simulink model "Demo_M1V4"  (R2015a)
settings: Solver=FixedStepDiscrete  SolverMode=SingleTasking  StartTime=0.0  StopTime=inf  FixedStep=.03  RelTol=1e-3
libraries: RASPlib x5, MinSegLibrary_M1V4 x4, arduinolib x3
settings Model: SimulationMode=external  ExtModeTrigDuration=2  Creator=Alec  LastModifiedBy=hurstj
settings OptimizationCC: ExpressionDepthLimit=2147483647  OptimizeModelRefInitCode=on  LifeSpan=1
settings DebuggingCC: UnderspecifiedInitializationDetection=Classic  MergeDetectMultiDrivingBlocksExec=none  StateNameClashWarn=warning
settings HardwareCC: ProdBitPerInt=16  ProdBitPerPointer=8  ProdIntDivRoundTo=Zero  ProdEndianess=LittleEndian  ProdWordSize=8  ProdHWDeviceType=Atmel->AVR
settings RTWCC: SystemTargetFile=realtime.tlc  GenerateMakefile=off  TemplateMakefile=realtime.tmf  Description=Real-Time Toolbox  RTWVerbose=off
settings CodeAppCC: CustomSymbolStrType=$N$R$M  InternalIdentifier=Classic
settings ERTTargetCC: CombineOutputUpdateFcns=off  ExtMode=on  ExtModeTransport=3  ExtModeMexArgs=0 6 115200  ERTSrcFileBannerTemplate=realtime_code_template.cgt  ERTHdrFileBannerTemplate=realtime_code_template.cgt  ERTDataSrcFileTemplate=realtime_code_template.cgt  ERTDataHdrFileTemplate=realtime_code_template.cgt  ERTCustomFileTemplate=realtime_file_process.tlc

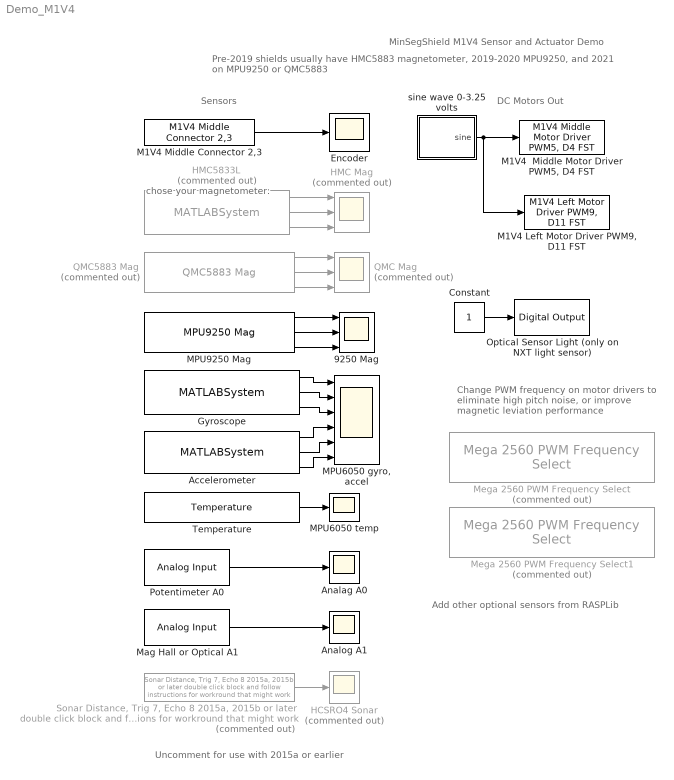
== system Demo_M1V4 ==
  note: Pre-2019 shields usually have HMC5883 magnetometer, 2019-2020 MPU9250,
      | and 2021 on MPU9250 or QMC5883
  note: chose your magnetometer:
  note: Add other optional sensors from RASPLib
  note: Uncomment for use with 2015a or earlier
  note: DC Motors Out
  note: Sensors
  note: MinSegShield M1V4 Sensor and Actuator Demo
  note: Change PWM frequency on motor drivers
      | to eliminate high pitch noise, or improve
      | magnetic leviation performance
  9250 Mag : Scope  NumInputPorts=3
      settings: TimeRange=30  YMin=-200~-200~-200  YMax=200~200~200  SaveName=ScopeData7  ScrollMode=on
  Accelerometer : MATLABSystem  System=soMPU6050Accel  SimulateUsing=Code generation
      mask Type: soMPU6050Accel
      mask Display:
      | disp('soMPU6050Accel');
      | port_label('output',1,'xaccel');
      | port_label('output',2,'yaccel');
      | port_label('output',3,'zaccel');
  Analag A0 : Scope
      settings: TimeRange=30  YMin=200  YMax=1100  SaveName=ScopeData6  ScrollMode=on
  Analog A1 : Scope
      settings: TimeRange=30  YMin=200  YMax=1100  SaveName=ScopeData3
  Constant : Constant
  Encoder : Scope
      settings: TimeRange=30  YMin=-1000  YMax=1000  ScrollMode=on
  Gyroscope : MATLABSystem  System=soMPU6050Gyro  DLPFmode=0
      mask Type: soMPU6050Gyro
      mask Display:
      | disp('soMPU6050Gyro');
      | port_label('output',1,'xvel');
      | port_label('output',2,'yvel');
      | port_label('output',3,'zvel');
  HCSRO4 Sonar : Scope  Commented=on
      settings: TimeRange=30  YMin=0  YMax=150  SaveName=ScopeData2
  HMC Mag : Scope  Commented=on  NumInputPorts=3
      settings: TimeRange=30  YMin=-200~-200~-200  YMax=200~200~200  SaveName=ScopeData4
  HMC5833L : MATLABSystem  Commented=on  System=soHMC5883L  SimulateUsing=Code generation
      mask Type: soHMC5883L
      mask Display:
      | disp('soHMC5883L');
      | port_label('output',1,'xmag');
      | port_label('output',2,'ymag');
      | port_label('output',3,'zmag');
  "M1V4  Middle Motor Driver PWM5, D4 FST" : MinSegLibrary_M1V4/M1V4  Middle Motor Driver PWM5, D4 FST  Vsupply=3.25
  "M1V4 Left Motor Driver PWM9, D11 FST" : MinSegLibrary_M1V4/M1V4 Left Motor Driver PWM9, D11 FST  Vsupply=3.25
  M1V4 Middle Connector 2,3 : MinSegLibrary_M1V4/M1V4 Middle Connector 2,3  Encoder=0  PinA=3  PinB=2
  "MPU6050 gyro, accel" : Scope  NumInputPorts=6
      settings: TimeRange=30  YMin=-30000~-30000~-30000~-15000~-15000~-15000  YMax=30000~30000~30000~15000~15000~30000  ScrollMode=on
  MPU6050 temp : Scope
      settings: TimeRange=30  YMin=-3750  YMax=-1750  SaveName=ScopeData5
  MPU9250 Mag : RASPlib/MPU9250 Mag  SimulateUsing=Code generation
  Mag Hall or Optical A1 : arduinolib/Analog Input  pinNumber=1  sampleTime=-1  blockPlatform=arduino
  Mega 2560 PWM Frequency Select : RASPlib/Mega 2560 PWM Frequency Select  Commented=on  Frequency=32KHz  Timer=2 - pins 9, 10
  Mega 2560 PWM Frequency Select1 : RASPlib/Mega 2560 PWM Frequency Select  Commented=on  Frequency=32KHz  Timer=3 - pins 2, 3, 5
  Optical Sensor Light (only on NXT light sensor) : arduinolib/Digital Output  pinNumber=12  blockPlatform=arduino
  Potentimeter A0 : arduinolib/Analog Input  pinNumber=0  sampleTime=-1  blockPlatform=arduino
  QMC Mag : Scope  Commented=on  NumInputPorts=3
      settings: TimeRange=30  YMin=-200~-200~-200  YMax=200~200~200  SaveName=ScopeData8
  QMC5883 Mag : RASPlib/QMC5883 Mag  Commented=on  SimulateUsing=Code generation
  "Sonar Distance, Trig 7, Echo 8 2015a, 2015b or later double click block and follow instructions for workround that might work" : MinSegLibrary_M1V4/Sonar Distance, Trig 7, Echo 8 2015a, 2015b or later double click block and follow instructions for workround that might work  Commented=on  Sonar=1  TrigPin=7  EchoPin=8
  Temperature : RASPlib/Temperature  SimulateUsing=Code generation
  sine wave 0-3.25 volts : Subsystem
  wires:
  sine wave 0-3.25 volts/1(sine) -> "M1V4 Left Motor Driver PWM9, D11 FST"/1, "M1V4  Middle Motor Driver PWM5, D4 FST"/1
  Potentimeter A0/1 -> Analag A0/1
  Mag Hall or Optical A1/1 -> Analog A1/1
  Constant/1 -> Optical Sensor Light (only on NXT light sensor)/1
  M1V4 Middle Connector 2,3/1 -> Encoder/1
  "Sonar Distance, Trig 7, Echo 8 2015a, 2015b or later double click block and follow instructions for workround that might work"/1 -> HCSRO4 Sonar/1
  Gyroscope/1 -> "MPU6050 gyro, accel"/1
  Gyroscope/2 -> "MPU6050 gyro, accel"/2
  Gyroscope/3 -> "MPU6050 gyro, accel"/3
  Accelerometer/1 -> "MPU6050 gyro, accel"/4
  Accelerometer/2 -> "MPU6050 gyro, accel"/5
  Accelerometer/3 -> "MPU6050 gyro, accel"/6
  HMC5833L/1 -> HMC Mag/1
  HMC5833L/2 -> HMC Mag/2
  HMC5833L/3 -> HMC Mag/3
  Temperature/1 -> MPU6050 temp/1
  MPU9250 Mag/2 -> 9250 Mag/2
  MPU9250 Mag/3 -> 9250 Mag/3
  MPU9250 Mag/1 -> 9250 Mag/1
  QMC5883 Mag/1 -> QMC Mag/1
  QMC5883 Mag/2 -> QMC Mag/2
  QMC5883 Mag/3 -> QMC Mag/3

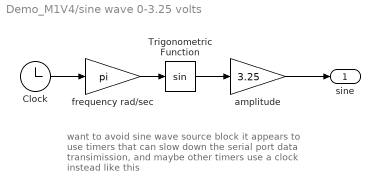
== system Demo_M1V4/sine wave 0-3.25 volts ==
  note: want to avoid sine wave source block
      | it appears to use timers that can slow down the
      | serial port data transimission, and maybe
      | other timers
      |
      | use a clock instead like this
  Clock : Clock
  Trigonometric Function : Trigonometry
  amplitude : Gain  Gain=3.25
  frequency rad/sec : Gain  Gain=pi
  sine : Outport
  wires:
  Clock/1 -> frequency rad/sec/1
  Trigonometric Function/1 -> amplitude/1
  frequency rad/sec/1 -> Trigonometric Function/1
  amplitude/1 -> sine/1
